simulink model "DirectionFinder"  (R2022b)
settings: Solver=VariableStepAuto  StartTime=0.0  StopTime=GV.SimTime  FixedStep=Pulse/2  RelTol=1e-3
values from neighbouring files (symbols this model uses):
  GV = GlobalVar    [RunDirectionFinder.m]
undefined symbols (not defined in the file or in its folder): S
libraries: dspswit3 x15, simrfV2elements x9, simrfV2util1 x9, dspstat3 x4, spsBistableLib x2, commrflib2 x2
settings Model: Creator=1NR_Operator_34  LastModifiedBy=1NR_Operator_34

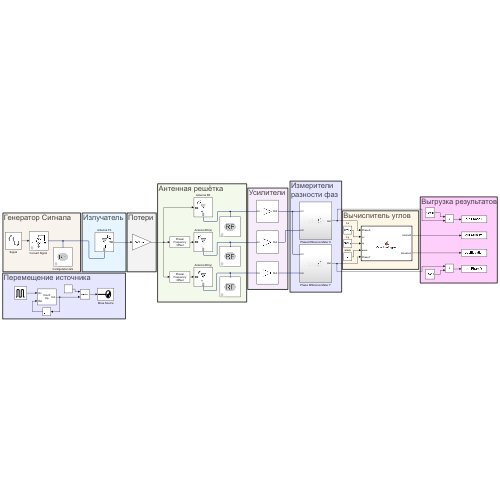
[thumbnail: Simulink's stored preview of the top-level diagram]
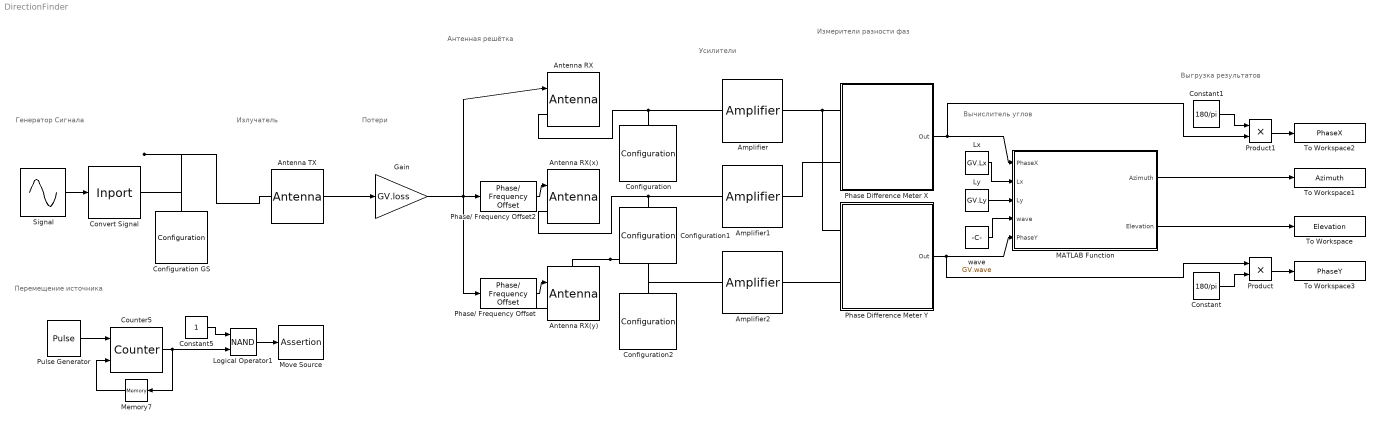
== system DirectionFinder ==
  note: Перемещение источника
  note: Измерители
      | разности фаз
  note: Антенная решётка
  note: Потери
  note: Излучатель
  note: Выгрузка результатов
  note: Вычислитель углов
  note: Усилители
  note: Генератор Сигнала
  Amplifier : simrfV2elements/Amplifier  classname=amplifier  DataSource=Data file  File=unitygain.s2p  isNetworkObj=off  Paramtype=S-parameters  Sparam=[0 0;1 0]  SparamFreq=1e9 Hz  SparamZ0=50  isRationalObj=off  Residues=0  Poles=0  DF={0 0; 1 0}  Source_linear_gain=Available power gain  linear_gain=GV.factor dB  AmAmAmPmTable=[-25,5,-1;-10,20,-2;0,27,5;5,28,12]  Zin=50  Zout=50  Source_Poly=Even and odd order  Poly_Coeffs=[0 1]  IPType=Output  IP2=inf dBm  IP3=inf dBm  P1dB=inf dBm  Psat=inf dBm  Gcomp=inf dBm  InternalGrounding=on  SourceFreq=Extracted from data source  PlotFreq=[1e9:1e6:3e9] Hz  PlotType=X-Y plane  YParam1=S(1,1)  YFormat1=Magnitude (dB)  YParam2=None  YFormat2=Magnitude (dB)  YOption=Linear  XOption=Linear  SparamRepresentation=Time domain (rationalfit)  FitTol=-40  FitOpt=Fit individually  MaxPoles=48  AutoImpulseLength=on  ImpulseLength=1e-10 s  MagModeling=off  AddNoise=on  NoiseType=Noise figure  NoiseDist=White  NF=0  MinNF=0  Gopt=0  RN=0  CarrierFreq=0 Hz  NoiseAutoImpulseLength=on  NoiseImpulseLength=1e-10 s  ConstS21NL=off  OpFreq=1 GHz  SetOpFreqAsMaxS21=off
  Amplifier1 : simrfV2elements/Amplifier  classname=amplifier  DataSource=Data file  File=unitygain.s2p  isNetworkObj=off  Paramtype=S-parameters  Sparam=[0 0;1 0]  SparamFreq=1e9 Hz  SparamZ0=50  isRationalObj=off  Residues=0  Poles=0  DF={0 0; 1 0}  Source_linear_gain=Available power gain  linear_gain=GV.factor dB  AmAmAmPmTable=[-25,5,-1;-10,20,-2;0,27,5;5,28,12]  Zin=50  Zout=50  Source_Poly=Even and odd order  Poly_Coeffs=[0 1]  IPType=Output  IP2=inf dBm  IP3=inf dBm  P1dB=inf dBm  Psat=inf dBm  Gcomp=inf dBm  InternalGrounding=on  SourceFreq=Extracted from data source  PlotFreq=[1e9:1e6:3e9] Hz  PlotType=X-Y plane  YParam1=S(1,1)  YFormat1=Magnitude (dB)  YParam2=None  YFormat2=Magnitude (dB)  YOption=Linear  XOption=Linear  SparamRepresentation=Time domain (rationalfit)  FitTol=-40  FitOpt=Fit individually  MaxPoles=48  AutoImpulseLength=on  ImpulseLength=1e-10 s  MagModeling=off  AddNoise=on  NoiseType=Noise figure  NoiseDist=White  NF=0  MinNF=0  Gopt=0  RN=0  CarrierFreq=0 Hz  NoiseAutoImpulseLength=on  NoiseImpulseLength=1e-10 s  ConstS21NL=off  OpFreq=1 GHz  SetOpFreqAsMaxS21=off
  Amplifier2 : simrfV2elements/Amplifier  classname=amplifier  DataSource=Data file  File=unitygain.s2p  isNetworkObj=off  Paramtype=S-parameters  Sparam=[0 0;1 0]  SparamFreq=1e9 Hz  SparamZ0=50  isRationalObj=off  Residues=0  Poles=0  DF={0 0; 1 0}  Source_linear_gain=Available power gain  linear_gain=GV.factor dB  AmAmAmPmTable=[-25,5,-1;-10,20,-2;0,27,5;5,28,12]  Zin=50  Zout=50  Source_Poly=Even and odd order  Poly_Coeffs=[0 1]  IPType=Output  IP2=inf dBm  IP3=inf dBm  P1dB=inf dBm  Psat=inf dBm  Gcomp=inf dBm  InternalGrounding=on  SourceFreq=Extracted from data source  PlotFreq=[1e9:1e6:3e9] Hz  PlotType=X-Y plane  YParam1=S(1,1)  YFormat1=Magnitude (dB)  YParam2=None  YFormat2=Magnitude (dB)  YOption=Linear  XOption=Linear  SparamRepresentation=Time domain (rationalfit)  FitTol=-40  FitOpt=Fit individually  MaxPoles=48  AutoImpulseLength=on  ImpulseLength=1e-10 s  MagModeling=off  AddNoise=on  NoiseType=Noise figure  NoiseDist=White  NF=0  MinNF=0  Gopt=0  RN=0  CarrierFreq=0 Hz  NoiseAutoImpulseLength=on  NoiseImpulseLength=1e-10 s  ConstS21NL=off  OpFreq=1 GHz  SetOpFreqAsMaxS21=off
  Antenna RX : simrfV2elements/Antenna  AntennaSource=Isotropic radiator  PrevAppliedAntSource=Isotropic radiator  Gr=5 dBi  Zin=50  AntennaObj=AntennaTX  InputIncWave=on  OutputRadWave=off  CarrierFreqInc=GV.freq Hz  rArr=[180 0] deg  CarrierFreqRad=10 Hz  rDep=[0 0] deg  AddNoise=on  InternalGrounding=on  SparamRepresentationImp=Time domain (rationalfit)  FitTolImp=-1  AutoImpulseLengthImp=on  ImpulseLengthImp=1e-10 s
  Antenna RX(x) : simrfV2elements/Antenna  AntennaSource=Isotropic radiator  PrevAppliedAntSource=Isotropic radiator  Gr=5 dBi  Zin=50  AntennaObj=AntennaTX  InputIncWave=on  OutputRadWave=off  CarrierFreqInc=GV.freq Hz  rArr=[180 0] deg  CarrierFreqRad=10 Hz  rDep=[0 0] deg  AddNoise=on  InternalGrounding=on  SparamRepresentationImp=Time domain (rationalfit)  FitTolImp=-1  AutoImpulseLengthImp=on  ImpulseLengthImp=1e-10 s
  Antenna RX(y) : simrfV2elements/Antenna  AntennaSource=Isotropic radiator  PrevAppliedAntSource=Isotropic radiator  Gr=5 dBi  Zin=50  AntennaObj=AntennaTX  InputIncWave=on  OutputRadWave=off  CarrierFreqInc=GV.freq Hz  rArr=[180 0] deg  CarrierFreqRad=10 Hz  rDep=[0 0] deg  AddNoise=on  InternalGrounding=on  SparamRepresentationImp=Time domain (rationalfit)  FitTolImp=-1  AutoImpulseLengthImp=on  ImpulseLengthImp=1e-10 s
  Antenna TX : simrfV2elements/Antenna  AntennaSource=Isotropic radiator  PrevAppliedAntSource=Isotropic radiator  Gr=5 dBi  Zin=50  AntennaObj=AntennaTX  InputIncWave=off  OutputRadWave=on  CarrierFreqInc=2.1 GHz  rArr=[180 0] deg  CarrierFreqRad=GV.freq Hz  rDep=[0 0] deg  AddNoise=on  InternalGrounding=on  SparamRepresentationImp=Time domain (rationalfit)  FitTolImp=-1  AutoImpulseLengthImp=on  ImpulseLengthImp=1e-10 s
  Configuration : simrfV2util1/Configuration  AutoFreq=on  Tones=[433] MHz  Harmonics=[7]  NormalizeCarrierPower=on  SolverType=Auto  UseCCode=on  StepSize=GV.SimStep s  AddNoise=on  defaultRNG=on  Seed=0  Temperature=290.0 K  SolverDelFlag=0  AbsTol=1e-6  RelTol=1e-3  MaxIter=10  ErrorEstimationType=2-norm over all variables  EnableInterpFilter=on  HiddenFIRfilterControllerParam=on  SmallSignalApprox=off  AllSimFreqs=on  SimFreqs=[] Hz  SimFreqsInternal=[]  SamplesPerFrame=1
  Configuration GS : simrfV2util1/Configuration  AutoFreq=on  Tones=[433] MHz  Harmonics=[7]  NormalizeCarrierPower=on  SolverType=Auto  UseCCode=on  StepSize=GV.SimStep s  AddNoise=on  defaultRNG=on  Seed=0  Temperature=290.0 K  SolverDelFlag=0  AbsTol=1e-6  RelTol=1e-3  MaxIter=10  ErrorEstimationType=2-norm over all variables  EnableInterpFilter=on  HiddenFIRfilterControllerParam=on  SmallSignalApprox=off  AllSimFreqs=on  SimFreqs=[] Hz  SimFreqsInternal=[]  SamplesPerFrame=1
  Configuration1 : simrfV2util1/Configuration  AutoFreq=on  Tones=[433] MHz  Harmonics=[7]  NormalizeCarrierPower=on  SolverType=Auto  UseCCode=on  StepSize=GV.SimStep s  AddNoise=on  defaultRNG=on  Seed=0  Temperature=290.0 K  SolverDelFlag=0  AbsTol=1e-6  RelTol=1e-3  MaxIter=10  ErrorEstimationType=2-norm over all variables  EnableInterpFilter=on  HiddenFIRfilterControllerParam=on  SmallSignalApprox=off  AllSimFreqs=on  SimFreqs=[] Hz  SimFreqsInternal=[]  SamplesPerFrame=1
  Configuration2 : simrfV2util1/Configuration  AutoFreq=on  Tones=[433] MHz  Harmonics=[7]  NormalizeCarrierPower=on  SolverType=Auto  UseCCode=on  StepSize=GV.SimStep s  AddNoise=on  defaultRNG=on  Seed=0  Temperature=290.0 K  SolverDelFlag=0  AbsTol=1e-6  RelTol=1e-3  MaxIter=10  ErrorEstimationType=2-norm over all variables  EnableInterpFilter=on  HiddenFIRfilterControllerParam=on  SmallSignalApprox=off  AllSimFreqs=on  SimFreqs=[] Hz  SimFreqsInternal=[]  SamplesPerFrame=1
  Constant : Constant  Value=180/pi
  Constant1 : Constant  Value=180/pi
  Constant5 : Constant
  "Convert Signal " : simrfV2util1/Inport  SimulinkInputSignalType=Ideal voltage  CarrierFreq=GV.freq Hz  ZS=0  UseSqWave=off  NumCoeff=10  Bias=0  DutyCyc=50  InternalGrounding=on
  Counter5 : dspswit3/Counter  Direction=Up  CountEvent=Rising edge  CounterSize=User defined  MaxCount=1  InitialCount=0  Output=Count  HitValue=32  ResetInput=on  SamplesPerFrame=1  Ts=1  CntDtype=double  HitDtype=Logical
  Gain : Gain  Gain=GV.loss
  Logical Operator1 : Logic  Operator=NAND  AllPortsSameDT=off  OutDataTypeStr=boolean
  Lx : Constant  Value=GV.Lx
  Ly : Constant  Value=GV.Ly
  MATLAB Function : MATLAB Function  TreatAsAtomicUnit=on
  Memory7 : Memory
  Move Source : Assertion  AssertionFailFcn=MoveSource  StopWhenAssertionFail=off
  Phase Difference Meter X : Subsystem
  Phase Difference Meter Y : Subsystem
  Phase/ Frequency Offset : commrflib2/Phase// Frequency Offset  phaseOffset=GV.PhaseY(GV.MoveStep)  freqPort=off  freqOffset=0
  Phase/ Frequency Offset2 : commrflib2/Phase// Frequency Offset  phaseOffset=GV.PhaseX(GV.MoveStep)  freqPort=off  freqOffset=0
  Product : Product
  Product1 : Product
  Pulse Generator : DiscretePulseGenerator  PulseType=Time based  Period=GV.SimTime  PulseWidth=50
  Signal : Sin  Amplitude=30  Frequency=2*pi*GV.freq  SampleTime=GV.SimStep
  To Workspace : ToWorkspace  VariableName=Elevation  SampleTime=GV.Measure
      settings: Save2DSignal=2-D array (concatenate along first dimension)
  To Workspace1 : ToWorkspace  VariableName=Azimuth  SampleTime=GV.Measure
      settings: Save2DSignal=2-D array (concatenate along first dimension)
  To Workspace2 : ToWorkspace  VariableName=PhaseX  SampleTime=GV.Measure
      settings: Save2DSignal=2-D array (concatenate along first dimension)
  To Workspace3 : ToWorkspace  VariableName=PhaseY  SampleTime=GV.Measure
      settings: Save2DSignal=2-D array (concatenate along first dimension)
  wave : Constant  Value=GV.wave
  wires:
  Antenna TX/1 -> Gain/1
  MATLAB Function/1(Azimuth) -> To Workspace1/1
  MATLAB Function/2(Elevation) -> To Workspace/1
  Product/1 -> To Workspace3/1
  Constant/1 -> Product/2
  Product1/1 -> To Workspace2/1
  Constant1/1 -> Product1/1
  Phase Difference Meter X/1(Out) -> Product1/2, MATLAB Function/1(PhaseX)
  Phase Difference Meter Y/1(Out) -> MATLAB Function/5(PhaseY), Product/1
  Signal/1 -> "Convert Signal "/1
  Lx/1 -> MATLAB Function/2(Lx)
  Ly/1 -> MATLAB Function/3(Ly)
  wave/1 -> MATLAB Function/4(wave)
  Pulse Generator/1 -> Counter5/1
  Counter5/1 -> Memory7/1, Logical Operator1/2
  Memory7/1 -> Counter5/2
  Constant5/1 -> Logical Operator1/1
  Logical Operator1/1 -> Move Source/1
  Gain/1 -> Antenna RX/1, Phase/ Frequency Offset2/1, Phase/ Frequency Offset/1
  Phase/ Frequency Offset/1 -> Antenna RX(y)/1
  Phase/ Frequency Offset2/1 -> Antenna RX(x)/1
  connections:
  Antenna TX/LConn1 -- "Convert Signal "/RConn1 -- Configuration GS/LConn1
  Amplifier/RConn1 -- Phase Difference Meter Y/LConn1 -- Phase Difference Meter X/LConn1
  Phase Difference Meter X/LConn2 -- Amplifier1/RConn1
  Phase Difference Meter Y/LConn2 -- Amplifier2/RConn1
  Antenna RX(y)/LConn1 -- Amplifier2/LConn1 -- Configuration2/LConn1
  Configuration1/LConn1 -- Amplifier1/LConn1 -- Antenna RX(x)/LConn1
  Configuration/LConn1 -- Amplifier/LConn1 -- Antenna RX/LConn1

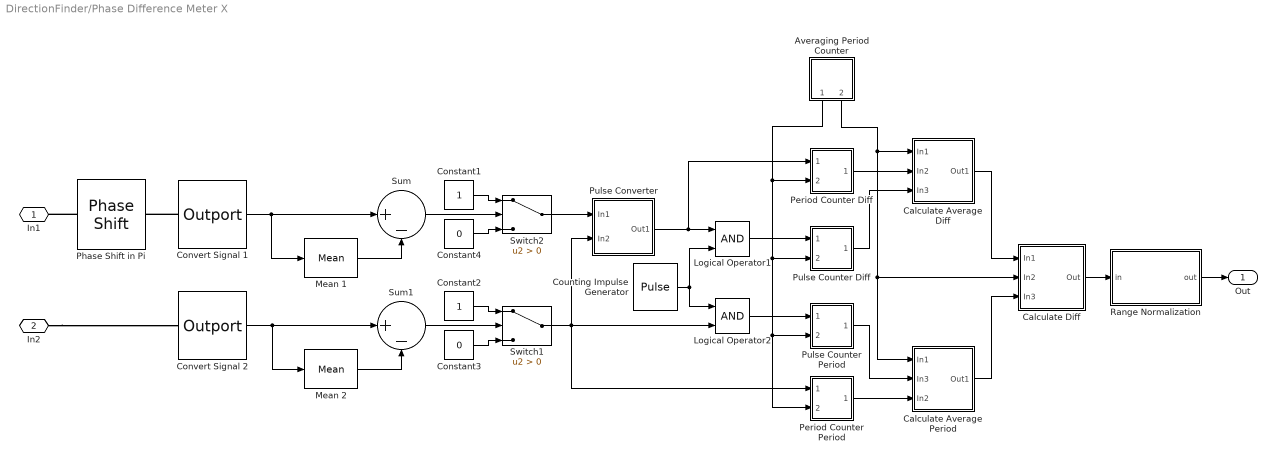
== system DirectionFinder/Phase Difference Meter X ==
  Averaging Period Counter : Subsystem
  Calculate Average Diff : Subsystem
  Calculate Average Period : Subsystem
  Calculate Diff : Subsystem
  Constant1 : Constant
  Constant2 : Constant
  Constant3 : Constant  Value=0
  Constant4 : Constant  Value=0
  Convert Signal 1 : simrfV2util1/Outport  SensorType=Ideal voltage  OutputFormat=Real Passband  CarrierFreq=GV.freq Hz  ZL=Inf  InternalGrounding=on  StepSize=2.3095e-12 s  AutoStep=on
  Convert Signal 2 : simrfV2util1/Outport  SensorType=Ideal voltage  OutputFormat=Real Passband  CarrierFreq=GV.freq Hz  ZL=Inf  InternalGrounding=on  StepSize=2.3095e-12 s  AutoStep=on
  Counting Impulse Generator : DiscretePulseGenerator  PulseType=Time based  Period=GV.Impulse  PulseWidth=50
  Logical Operator1 : Logic  AllPortsSameDT=off  OutDataTypeStr=boolean
  Logical Operator2 : Logic  AllPortsSameDT=off  OutDataTypeStr=boolean
  Mean 1 : dspstat3/Mean  run=on  InputProcessing=Columns as channels (frame based)  reset_popup=None  directionMode=Each column  dimension=1  roiEnable=off  roiType=Rectangles  roiPortion=Entire ROI  roiOutput=Individual statistics for each ROI  roiFlag=off  roundingMode=Floor  overflowMode=off  outputDataTypeStr=Inherit: Same as accumulator  outputMin=[]  outputMax=[]  outputLastDataTypeStr=Inherit: Same as accumulator
  Mean 2 : dspstat3/Mean  run=on  InputProcessing=Columns as channels (frame based)  reset_popup=None  directionMode=Each column  dimension=1  roiEnable=off  roiType=Rectangles  roiPortion=Entire ROI  roiOutput=Individual statistics for each ROI  roiFlag=off  roundingMode=Floor  overflowMode=off  outputDataTypeStr=Inherit: Same as accumulator  outputMin=[]  outputMax=[]  outputLastDataTypeStr=Inherit: Same as accumulator
  Period Counter Diff : Subsystem
  Period Counter Period : Subsystem
  Phase Shift in Pi : simrfV2elements/Phase Shift  PhaseShift=180 deg  InternalGrounding=on
  Pulse Converter : Subsystem
  Pulse Counter Diff : Subsystem
  Pulse Counter Period : Subsystem
  Range Normalization : MATLAB Function  TreatAsAtomicUnit=on
  Sum : Sum  Inputs=|+-
  Sum1 : Sum  Inputs=|+-
  Switch1 : Switch  Criteria=u2 > Threshold  SaturateOnIntegerOverflow=off  InputSameDT=off
  Switch2 : Switch  Criteria=u2 > Threshold  SaturateOnIntegerOverflow=off  InputSameDT=off
  In1 : PMIOPort  Side=Left
  In2 : PMIOPort  Port=2  Side=Left
  Out : Outport
  wires:
  Period Counter Diff/1(Out1) -> Calculate Average Diff/2(In2)
  Averaging Period Counter/1(Out1) -> Period Counter Period/2(In2), Pulse Counter Period/2(In2), Pulse Counter Diff/2(In2), Period Counter Diff/2(In2)
  Sum1/1 -> Switch1/2
  Calculate Average Period/1(Out1) -> Calculate Diff/3(In3)
  Pulse Counter Period/1(Out1) -> Calculate Average Period/2(In3)
  Counting Impulse Generator/1 -> Logical Operator1/2, Logical Operator2/1
  Mean 2/1 -> Sum1/2
  Convert Signal 1/1 -> Mean 1/1, Sum/1
  Mean 1/1 -> Sum/2
  Pulse Counter Diff/1(Out1) -> Calculate Average Diff/3(In3)
  Averaging Period Counter/2(Out2) -> Calculate Average Period/1(In1), Calculate Diff/2(In2), Calculate Average Diff/1(In1)
  Convert Signal 2/1 -> Mean 2/1, Sum1/1
  Logical Operator1/1 -> Pulse Counter Diff/1(In1)
  Calculate Average Diff/1(Out1) -> Calculate Diff/1(In1)
  Period Counter Period/1(Out1) -> Calculate Average Period/3(In2)
  Logical Operator2/1 -> Pulse Counter Period/1(In1)
  Switch2/1 -> Pulse Converter/1(In1)
  Switch1/1 -> Logical Operator2/2, Period Counter Period/1(In1), Pulse Converter/2(In2)
  Pulse Converter/1(Out1) -> Logical Operator1/1, Period Counter Diff/1(In1)
  Calculate Diff/1(Out) -> Range Normalization/1(in)
  Range Normalization/1(out) -> Out/1
  Constant2/1 -> Switch1/1
  Constant3/1 -> Switch1/3
  Sum/1 -> Switch2/2
  Constant1/1 -> Switch2/1
  Constant4/1 -> Switch2/3
  connections:
  In2/RConn1 -- Convert Signal 2/LConn1
  Convert Signal 1/LConn1 -- Phase Shift in Pi/RConn1
  Phase Shift in Pi/LConn1 -- In1/RConn1

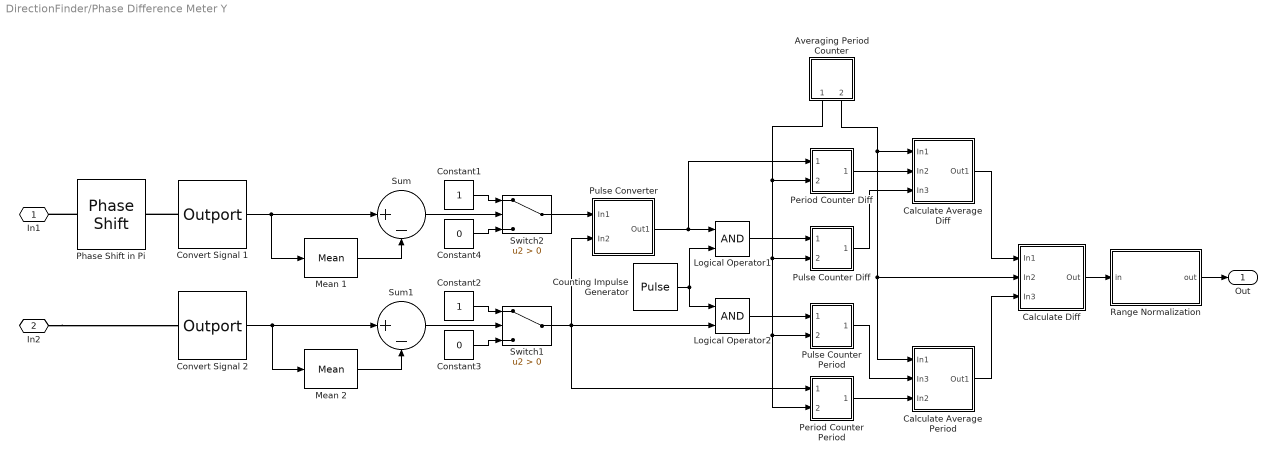
== system DirectionFinder/Phase Difference Meter Y ==
  Averaging Period Counter : Subsystem
  Calculate Average Diff : Subsystem
  Calculate Average Period : Subsystem
  Calculate Diff : Subsystem
  Constant1 : Constant
  Constant2 : Constant
  Constant3 : Constant  Value=0
  Constant4 : Constant  Value=0
  Convert Signal 1 : simrfV2util1/Outport  SensorType=Ideal voltage  OutputFormat=Real Passband  CarrierFreq=GV.freq Hz  ZL=Inf  InternalGrounding=on  StepSize=2.3095e-12 s  AutoStep=on
  Convert Signal 2 : simrfV2util1/Outport  SensorType=Ideal voltage  OutputFormat=Real Passband  CarrierFreq=GV.freq Hz  ZL=Inf  InternalGrounding=on  StepSize=2.3095e-12 s  AutoStep=on
  Counting Impulse Generator : DiscretePulseGenerator  PulseType=Time based  Period=GV.Impulse  PulseWidth=50
  Logical Operator1 : Logic  AllPortsSameDT=off  OutDataTypeStr=boolean
  Logical Operator2 : Logic  AllPortsSameDT=off  OutDataTypeStr=boolean
  Mean 1 : dspstat3/Mean  run=on  InputProcessing=Columns as channels (frame based)  reset_popup=None  directionMode=Each column  dimension=1  roiEnable=off  roiType=Rectangles  roiPortion=Entire ROI  roiOutput=Individual statistics for each ROI  roiFlag=off  roundingMode=Floor  overflowMode=off  outputDataTypeStr=Inherit: Same as accumulator  outputMin=[]  outputMax=[]  outputLastDataTypeStr=Inherit: Same as accumulator
  Mean 2 : dspstat3/Mean  run=on  InputProcessing=Columns as channels (frame based)  reset_popup=None  directionMode=Each column  dimension=1  roiEnable=off  roiType=Rectangles  roiPortion=Entire ROI  roiOutput=Individual statistics for each ROI  roiFlag=off  roundingMode=Floor  overflowMode=off  outputDataTypeStr=Inherit: Same as accumulator  outputMin=[]  outputMax=[]  outputLastDataTypeStr=Inherit: Same as accumulator
  Period Counter Diff : Subsystem
  Period Counter Period : Subsystem
  Phase Shift in Pi : simrfV2elements/Phase Shift  PhaseShift=180 deg  InternalGrounding=on
  Pulse Converter : Subsystem
  Pulse Counter Diff : Subsystem
  Pulse Counter Period : Subsystem
  Range Normalization : MATLAB Function  TreatAsAtomicUnit=on
  Sum : Sum  Inputs=|+-
  Sum1 : Sum  Inputs=|+-
  Switch1 : Switch  Criteria=u2 > Threshold  SaturateOnIntegerOverflow=off  InputSameDT=off
  Switch2 : Switch  Criteria=u2 > Threshold  SaturateOnIntegerOverflow=off  InputSameDT=off
  In1 : PMIOPort  Side=Left
  In2 : PMIOPort  Port=2  Side=Left
  Out : Outport
  wires:
  Period Counter Diff/1(Out1) -> Calculate Average Diff/2(In2)
  Averaging Period Counter/1(Out1) -> Period Counter Period/2(In2), Pulse Counter Period/2(In2), Pulse Counter Diff/2(In2), Period Counter Diff/2(In2)
  Sum1/1 -> Switch1/2
  Calculate Average Period/1(Out1) -> Calculate Diff/3(In3)
  Pulse Counter Period/1(Out1) -> Calculate Average Period/2(In3)
  Counting Impulse Generator/1 -> Logical Operator1/2, Logical Operator2/1
  Mean 2/1 -> Sum1/2
  Convert Signal 1/1 -> Mean 1/1, Sum/1
  Mean 1/1 -> Sum/2
  Pulse Counter Diff/1(Out1) -> Calculate Average Diff/3(In3)
  Averaging Period Counter/2(Out2) -> Calculate Average Period/1(In1), Calculate Diff/2(In2), Calculate Average Diff/1(In1)
  Convert Signal 2/1 -> Mean 2/1, Sum1/1
  Logical Operator1/1 -> Pulse Counter Diff/1(In1)
  Calculate Average Diff/1(Out1) -> Calculate Diff/1(In1)
  Period Counter Period/1(Out1) -> Calculate Average Period/3(In2)
  Logical Operator2/1 -> Pulse Counter Period/1(In1)
  Switch2/1 -> Pulse Converter/1(In1)
  Switch1/1 -> Logical Operator2/2, Period Counter Period/1(In1), Pulse Converter/2(In2)
  Pulse Converter/1(Out1) -> Logical Operator1/1, Period Counter Diff/1(In1)
  Calculate Diff/1(Out) -> Range Normalization/1(in)
  Range Normalization/1(out) -> Out/1
  Constant2/1 -> Switch1/1
  Constant3/1 -> Switch1/3
  Sum/1 -> Switch2/2
  Constant1/1 -> Switch2/1
  Constant4/1 -> Switch2/3
  connections:
  In2/RConn1 -- Convert Signal 2/LConn1
  Convert Signal 1/LConn1 -- Phase Shift in Pi/RConn1
  Phase Shift in Pi/LConn1 -- In1/RConn1

== system DirectionFinder/Phase Difference Meter X/Averaging Period Counter ==
  Constant1 : Constant
  Counter6 : dspswit3/Counter  Direction=Up  CountEvent=Rising edge  CounterSize=User defined  MaxCount=1  InitialCount=0  Output=Count  HitValue=32  ResetInput=on  SamplesPerFrame=1  Ts=1  CntDtype=double  HitDtype=Logical
  Delay : Delay  DelayLength=1  InitialCondition=0
  Logical Operator7 : Logic  Operator=NAND  AllPortsSameDT=off  OutDataTypeStr=boolean
  Measure Period Generator : DiscretePulseGenerator  PulseType=Time based  Period=GV.Measure  PulseWidth=50
  Memory : Memory
  Out1 : Outport
  Out2 : Outport  Port=2
  wires:
  Delay/1 -> Out1/1
  Logical Operator7/1 -> Delay/1
  Measure Period Generator/1 -> Counter6/1
  Counter6/1 -> Memory/1, Out2/1, Logical Operator7/2
  Memory/1 -> Counter6/2
  Constant1/1 -> Logical Operator7/1

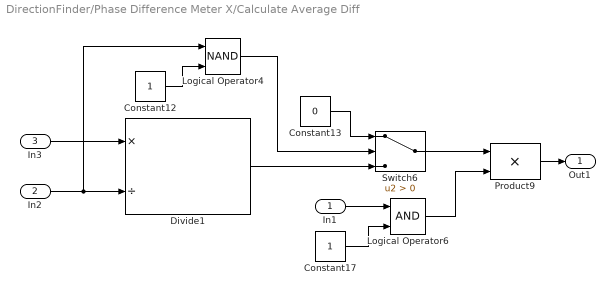
== system DirectionFinder/Phase Difference Meter X/Calculate Average Diff ==
  In1 : Inport
  In2 : Inport  Port=2
  In3 : Inport  Port=3
  Constant12 : Constant
  Constant13 : Constant  Value=0
  Constant17 : Constant
  Divide1 : Product  Inputs=*/
  Logical Operator4 : Logic  Operator=NAND  AllPortsSameDT=off  OutDataTypeStr=boolean
  Logical Operator6 : Logic  AllPortsSameDT=off  OutDataTypeStr=boolean
  Product9 : Product
  Switch6 : Switch  Criteria=u2 > Threshold  SaturateOnIntegerOverflow=off  InputSameDT=off
  Out1 : Outport
  wires:
  Divide1/1 -> Switch6/3
  Logical Operator6/1 -> Product9/2
  Constant17/1 -> Logical Operator6/2
  Constant12/1 -> Logical Operator4/2
  Logical Operator4/1 -> Switch6/2
  Constant13/1 -> Switch6/1
  Switch6/1 -> Product9/1
  In2/1 -> Logical Operator4/1, Divide1/2
  Product9/1 -> Out1/1
  In1/1 -> Logical Operator6/1
  In3/1 -> Divide1/1

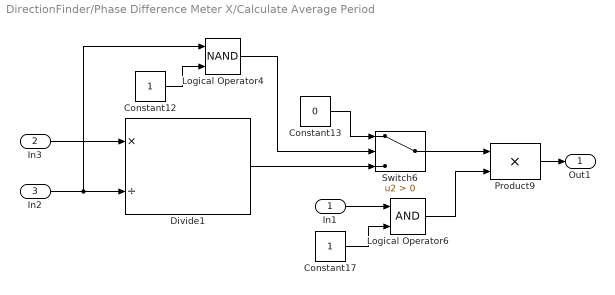
== system DirectionFinder/Phase Difference Meter X/Calculate Average Period ==
  In1 : Inport
  In3 : Inport  Port=2
  In2 : Inport  Port=3
  Constant12 : Constant
  Constant13 : Constant  Value=0
  Constant17 : Constant
  Divide1 : Product  Inputs=*/
  Logical Operator4 : Logic  Operator=NAND  AllPortsSameDT=off  OutDataTypeStr=boolean
  Logical Operator6 : Logic  AllPortsSameDT=off  OutDataTypeStr=boolean
  Product9 : Product
  Switch6 : Switch  Criteria=u2 > Threshold  SaturateOnIntegerOverflow=off  InputSameDT=off
  Out1 : Outport
  wires:
  Divide1/1 -> Switch6/3
  Logical Operator6/1 -> Product9/2
  Constant17/1 -> Logical Operator6/2
  Constant12/1 -> Logical Operator4/2
  Logical Operator4/1 -> Switch6/2
  Constant13/1 -> Switch6/1
  Switch6/1 -> Product9/1
  In2/1 -> Logical Operator4/1, Divide1/2
  Product9/1 -> Out1/1
  In1/1 -> Logical Operator6/1
  In3/1 -> Divide1/1

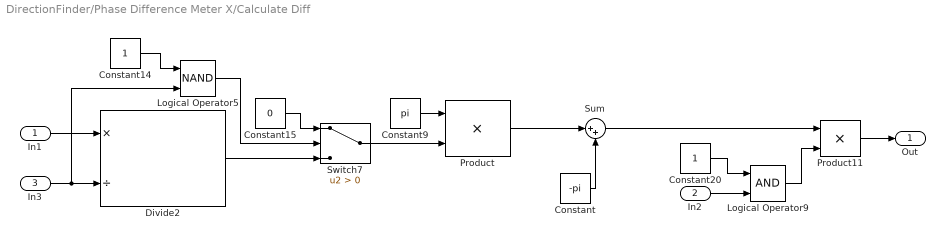
== system DirectionFinder/Phase Difference Meter X/Calculate Diff ==
  In1 : Inport
  In2 : Inport  Port=2
  In3 : Inport  Port=3
  Constant : Constant  Value=-pi
  Constant14 : Constant
  Constant15 : Constant  Value=0
  Constant20 : Constant
  Constant9 : Constant  Value=pi
  Divide2 : Product  Inputs=*/
  Logical Operator5 : Logic  Operator=NAND  AllPortsSameDT=off  OutDataTypeStr=boolean
  Logical Operator9 : Logic  AllPortsSameDT=off  OutDataTypeStr=boolean
  Product : Product
  Product11 : Product
  Sum : Sum  Inputs=|++
  Switch7 : Switch  Criteria=u2 > Threshold  SaturateOnIntegerOverflow=off  InputSameDT=off
  Out : Outport
  wires:
  Constant9/1 -> Product/1
  Divide2/1 -> Switch7/3
  Logical Operator5/1 -> Switch7/2
  In3/1 -> Logical Operator5/2, Divide2/2
  Switch7/1 -> Product/2
  Constant15/1 -> Switch7/1
  Logical Operator9/1 -> Product11/2
  Product11/1 -> Out/1
  In1/1 -> Divide2/1
  Constant14/1 -> Logical Operator5/1
  Constant20/1 -> Logical Operator9/1
  In2/1 -> Logical Operator9/2
  Constant/1 -> Sum/2
  Product/1 -> Sum/1
  Sum/1 -> Product11/1

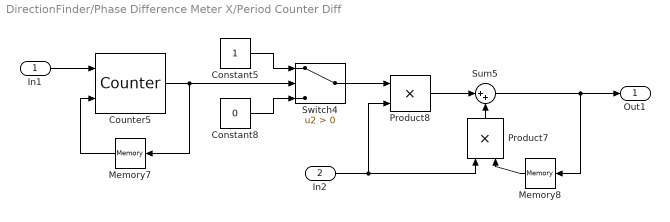
== system DirectionFinder/Phase Difference Meter X/Period Counter Diff ==
  In1 : Inport
  In2 : Inport  Port=2
  Constant5 : Constant
  Constant8 : Constant  Value=0
  Counter5 : dspswit3/Counter  Direction=Up  CountEvent=Rising edge  CounterSize=User defined  MaxCount=1  InitialCount=0  Output=Count  HitValue=32  ResetInput=on  SamplesPerFrame=1  Ts=1  CntDtype=double  HitDtype=Logical
  Memory7 : Memory
  Memory8 : Memory
  Product7 : Product
  Product8 : Product
  Sum5 : Sum  Inputs=|++
  Switch4 : Switch  Criteria=u2 > Threshold  SaturateOnIntegerOverflow=off  InputSameDT=off
  Out1 : Outport
  wires:
  Counter5/1 -> Memory7/1, Switch4/2
  Product8/1 -> Sum5/1
  Switch4/1 -> Product8/1
  Constant5/1 -> Switch4/1
  Sum5/1 -> Out1/1, Memory8/1
  Memory8/1 -> Product7/2
  Constant8/1 -> Switch4/3
  Memory7/1 -> Counter5/2
  In2/1 -> Product7/1, Product8/2
  Product7/1 -> Sum5/2
  In1/1 -> Counter5/1

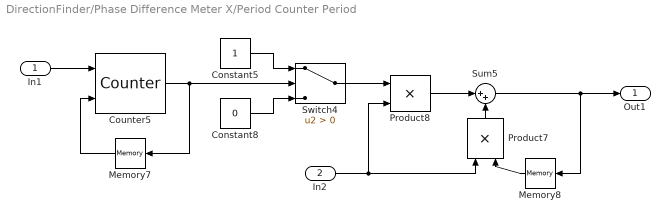
== system DirectionFinder/Phase Difference Meter X/Period Counter Period ==
  In1 : Inport
  In2 : Inport  Port=2
  Constant5 : Constant
  Constant8 : Constant  Value=0
  Counter5 : dspswit3/Counter  Direction=Up  CountEvent=Rising edge  CounterSize=User defined  MaxCount=1  InitialCount=0  Output=Count  HitValue=32  ResetInput=on  SamplesPerFrame=1  Ts=1  CntDtype=double  HitDtype=Logical
  Memory7 : Memory
  Memory8 : Memory
  Product7 : Product
  Product8 : Product
  Sum5 : Sum  Inputs=|++
  Switch4 : Switch  Criteria=u2 > Threshold  SaturateOnIntegerOverflow=off  InputSameDT=off
  Out1 : Outport
  wires:
  Counter5/1 -> Memory7/1, Switch4/2
  Product8/1 -> Sum5/1
  Switch4/1 -> Product8/1
  Constant5/1 -> Switch4/1
  Sum5/1 -> Out1/1, Memory8/1
  Memory8/1 -> Product7/2
  Constant8/1 -> Switch4/3
  Memory7/1 -> Counter5/2
  In2/1 -> Product7/1, Product8/2
  Product7/1 -> Sum5/2
  In1/1 -> Counter5/1

== system DirectionFinder/Phase Difference Meter X/Pulse Converter ==
  In1 : Inport
  In2 : Inport  Port=2
  Bistable : spsBistableLib/Bistable  Qpriority=Set  ic=0  Ts=0
      settings: LibrarySourceBlock=sps_lib/Control/Bistable
  Counter1 : dspswit3/Counter  Direction=Up  CountEvent=Rising edge  CounterSize=User defined  MaxCount=1  InitialCount=0  Output=Count  HitValue=32  ResetInput=on  SamplesPerFrame=1  Ts=1  CntDtype=double  HitDtype=Logical
  Counter5 : dspswit3/Counter  Direction=Up  CountEvent=Rising edge  CounterSize=User defined  MaxCount=1  InitialCount=0  Output=Count  HitValue=32  ResetInput=on  SamplesPerFrame=1  Ts=1  CntDtype=double  HitDtype=Logical
  Memory1 : Memory
  Memory7 : Memory
  Terminator : Terminator
  Out1 : Outport
  wires:
  Memory7/1 -> Counter5/2
  Counter5/1 -> Memory7/1, Bistable/1
  In1/1 -> Counter5/1
  In2/1 -> Counter1/1
  Counter1/1 -> Bistable/2, Memory1/1
  Memory1/1 -> Counter1/2
  Bistable/1 -> Terminator/1
  Bistable/2 -> Out1/1

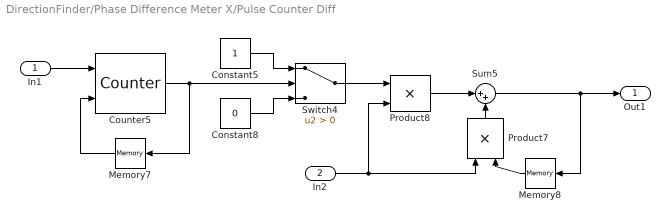
== system DirectionFinder/Phase Difference Meter X/Pulse Counter Diff ==
  In1 : Inport
  In2 : Inport  Port=2
  Constant5 : Constant
  Constant8 : Constant  Value=0
  Counter5 : dspswit3/Counter  Direction=Up  CountEvent=Rising edge  CounterSize=User defined  MaxCount=1  InitialCount=0  Output=Count  HitValue=32  ResetInput=on  SamplesPerFrame=1  Ts=1  CntDtype=double  HitDtype=Logical
  Memory7 : Memory
  Memory8 : Memory
  Product7 : Product
  Product8 : Product
  Sum5 : Sum  Inputs=|++
  Switch4 : Switch  Criteria=u2 > Threshold  SaturateOnIntegerOverflow=off  InputSameDT=off
  Out1 : Outport
  wires:
  Counter5/1 -> Memory7/1, Switch4/2
  Product8/1 -> Sum5/1
  Switch4/1 -> Product8/1
  Constant5/1 -> Switch4/1
  Sum5/1 -> Out1/1, Memory8/1
  Memory8/1 -> Product7/2
  Constant8/1 -> Switch4/3
  Memory7/1 -> Counter5/2
  In2/1 -> Product7/1, Product8/2
  Product7/1 -> Sum5/2
  In1/1 -> Counter5/1

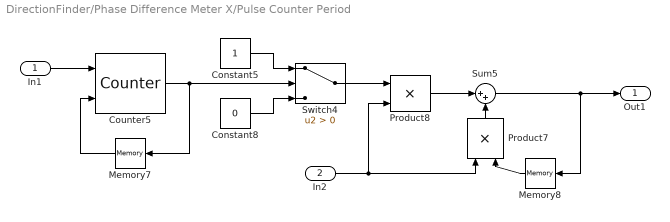
== system DirectionFinder/Phase Difference Meter X/Pulse Counter Period ==
  In1 : Inport
  In2 : Inport  Port=2
  Constant5 : Constant
  Constant8 : Constant  Value=0
  Counter5 : dspswit3/Counter  Direction=Up  CountEvent=Rising edge  CounterSize=User defined  MaxCount=1  InitialCount=0  Output=Count  HitValue=32  ResetInput=on  SamplesPerFrame=1  Ts=1  CntDtype=double  HitDtype=Logical
  Memory7 : Memory
  Memory8 : Memory
  Product7 : Product
  Product8 : Product
  Sum5 : Sum  Inputs=|++
  Switch4 : Switch  Criteria=u2 > Threshold  SaturateOnIntegerOverflow=off  InputSameDT=off
  Out1 : Outport
  wires:
  Counter5/1 -> Memory7/1, Switch4/2
  Product8/1 -> Sum5/1
  Switch4/1 -> Product8/1
  Constant5/1 -> Switch4/1
  Sum5/1 -> Out1/1, Memory8/1
  Memory8/1 -> Product7/2
  Constant8/1 -> Switch4/3
  Memory7/1 -> Counter5/2
  In2/1 -> Product7/1, Product8/2
  Product7/1 -> Sum5/2
  In1/1 -> Counter5/1

== system DirectionFinder/Phase Difference Meter Y/Averaging Period Counter ==
  Constant1 : Constant
  Counter6 : dspswit3/Counter  Direction=Up  CountEvent=Rising edge  CounterSize=User defined  MaxCount=1  InitialCount=0  Output=Count  HitValue=32  ResetInput=on  SamplesPerFrame=1  Ts=1  CntDtype=double  HitDtype=Logical
  Delay : Delay  DelayLength=1  InitialCondition=0
  Logical Operator7 : Logic  Operator=NAND  AllPortsSameDT=off  OutDataTypeStr=boolean
  Measure Period Generator : DiscretePulseGenerator  PulseType=Time based  Period=GV.Measure  PulseWidth=50
  Memory : Memory
  Out1 : Outport
  Out2 : Outport  Port=2
  wires:
  Delay/1 -> Out1/1
  Logical Operator7/1 -> Delay/1
  Measure Period Generator/1 -> Counter6/1
  Counter6/1 -> Memory/1, Out2/1, Logical Operator7/2
  Memory/1 -> Counter6/2
  Constant1/1 -> Logical Operator7/1

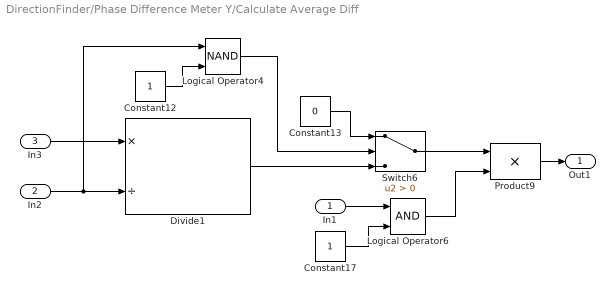
== system DirectionFinder/Phase Difference Meter Y/Calculate Average Diff ==
  In1 : Inport
  In2 : Inport  Port=2
  In3 : Inport  Port=3
  Constant12 : Constant
  Constant13 : Constant  Value=0
  Constant17 : Constant
  Divide1 : Product  Inputs=*/
  Logical Operator4 : Logic  Operator=NAND  AllPortsSameDT=off  OutDataTypeStr=boolean
  Logical Operator6 : Logic  AllPortsSameDT=off  OutDataTypeStr=boolean
  Product9 : Product
  Switch6 : Switch  Criteria=u2 > Threshold  SaturateOnIntegerOverflow=off  InputSameDT=off
  Out1 : Outport
  wires:
  Divide1/1 -> Switch6/3
  Logical Operator6/1 -> Product9/2
  Constant17/1 -> Logical Operator6/2
  Constant12/1 -> Logical Operator4/2
  Logical Operator4/1 -> Switch6/2
  Constant13/1 -> Switch6/1
  Switch6/1 -> Product9/1
  In2/1 -> Logical Operator4/1, Divide1/2
  Product9/1 -> Out1/1
  In1/1 -> Logical Operator6/1
  In3/1 -> Divide1/1

== system DirectionFinder/Phase Difference Meter Y/Calculate Average Period ==
  In1 : Inport
  In3 : Inport  Port=2
  In2 : Inport  Port=3
  Constant12 : Constant
  Constant13 : Constant  Value=0
  Constant17 : Constant
  Divide1 : Product  Inputs=*/
  Logical Operator4 : Logic  Operator=NAND  AllPortsSameDT=off  OutDataTypeStr=boolean
  Logical Operator6 : Logic  AllPortsSameDT=off  OutDataTypeStr=boolean
  Product9 : Product
  Switch6 : Switch  Criteria=u2 > Threshold  SaturateOnIntegerOverflow=off  InputSameDT=off
  Out1 : Outport
  wires:
  Divide1/1 -> Switch6/3
  Logical Operator6/1 -> Product9/2
  Constant17/1 -> Logical Operator6/2
  Constant12/1 -> Logical Operator4/2
  Logical Operator4/1 -> Switch6/2
  Constant13/1 -> Switch6/1
  Switch6/1 -> Product9/1
  In2/1 -> Logical Operator4/1, Divide1/2
  Product9/1 -> Out1/1
  In1/1 -> Logical Operator6/1
  In3/1 -> Divide1/1

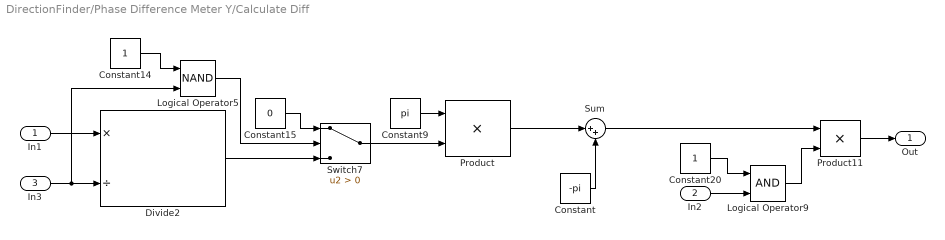
== system DirectionFinder/Phase Difference Meter Y/Calculate Diff ==
  In1 : Inport
  In2 : Inport  Port=2
  In3 : Inport  Port=3
  Constant : Constant  Value=-pi
  Constant14 : Constant
  Constant15 : Constant  Value=0
  Constant20 : Constant
  Constant9 : Constant  Value=pi
  Divide2 : Product  Inputs=*/
  Logical Operator5 : Logic  Operator=NAND  AllPortsSameDT=off  OutDataTypeStr=boolean
  Logical Operator9 : Logic  AllPortsSameDT=off  OutDataTypeStr=boolean
  Product : Product
  Product11 : Product
  Sum : Sum  Inputs=|++
  Switch7 : Switch  Criteria=u2 > Threshold  SaturateOnIntegerOverflow=off  InputSameDT=off
  Out : Outport
  wires:
  Constant9/1 -> Product/1
  Divide2/1 -> Switch7/3
  Logical Operator5/1 -> Switch7/2
  In3/1 -> Logical Operator5/2, Divide2/2
  Switch7/1 -> Product/2
  Constant15/1 -> Switch7/1
  Logical Operator9/1 -> Product11/2
  Product11/1 -> Out/1
  In1/1 -> Divide2/1
  Constant14/1 -> Logical Operator5/1
  Constant20/1 -> Logical Operator9/1
  In2/1 -> Logical Operator9/2
  Constant/1 -> Sum/2
  Product/1 -> Sum/1
  Sum/1 -> Product11/1

== system DirectionFinder/Phase Difference Meter Y/Period Counter Diff ==
  In1 : Inport
  In2 : Inport  Port=2
  Constant5 : Constant
  Constant8 : Constant  Value=0
  Counter5 : dspswit3/Counter  Direction=Up  CountEvent=Rising edge  CounterSize=User defined  MaxCount=1  InitialCount=0  Output=Count  HitValue=32  ResetInput=on  SamplesPerFrame=1  Ts=1  CntDtype=double  HitDtype=Logical
  Memory7 : Memory
  Memory8 : Memory
  Product7 : Product
  Product8 : Product
  Sum5 : Sum  Inputs=|++
  Switch4 : Switch  Criteria=u2 > Threshold  SaturateOnIntegerOverflow=off  InputSameDT=off
  Out1 : Outport
  wires:
  Counter5/1 -> Memory7/1, Switch4/2
  Product8/1 -> Sum5/1
  Switch4/1 -> Product8/1
  Constant5/1 -> Switch4/1
  Sum5/1 -> Out1/1, Memory8/1
  Memory8/1 -> Product7/2
  Constant8/1 -> Switch4/3
  Memory7/1 -> Counter5/2
  In2/1 -> Product7/1, Product8/2
  Product7/1 -> Sum5/2
  In1/1 -> Counter5/1

== system DirectionFinder/Phase Difference Meter Y/Period Counter Period ==
  In1 : Inport
  In2 : Inport  Port=2
  Constant5 : Constant
  Constant8 : Constant  Value=0
  Counter5 : dspswit3/Counter  Direction=Up  CountEvent=Rising edge  CounterSize=User defined  MaxCount=1  InitialCount=0  Output=Count  HitValue=32  ResetInput=on  SamplesPerFrame=1  Ts=1  CntDtype=double  HitDtype=Logical
  Memory7 : Memory
  Memory8 : Memory
  Product7 : Product
  Product8 : Product
  Sum5 : Sum  Inputs=|++
  Switch4 : Switch  Criteria=u2 > Threshold  SaturateOnIntegerOverflow=off  InputSameDT=off
  Out1 : Outport
  wires:
  Counter5/1 -> Memory7/1, Switch4/2
  Product8/1 -> Sum5/1
  Switch4/1 -> Product8/1
  Constant5/1 -> Switch4/1
  Sum5/1 -> Out1/1, Memory8/1
  Memory8/1 -> Product7/2
  Constant8/1 -> Switch4/3
  Memory7/1 -> Counter5/2
  In2/1 -> Product7/1, Product8/2
  Product7/1 -> Sum5/2
  In1/1 -> Counter5/1

== system DirectionFinder/Phase Difference Meter Y/Pulse Converter ==
  In1 : Inport
  In2 : Inport  Port=2
  Bistable : spsBistableLib/Bistable  Qpriority=Set  ic=0  Ts=0
      settings: LibrarySourceBlock=sps_lib/Control/Bistable
  Counter1 : dspswit3/Counter  Direction=Up  CountEvent=Rising edge  CounterSize=User defined  MaxCount=1  InitialCount=0  Output=Count  HitValue=32  ResetInput=on  SamplesPerFrame=1  Ts=1  CntDtype=double  HitDtype=Logical
  Counter5 : dspswit3/Counter  Direction=Up  CountEvent=Rising edge  CounterSize=User defined  MaxCount=1  InitialCount=0  Output=Count  HitValue=32  ResetInput=on  SamplesPerFrame=1  Ts=1  CntDtype=double  HitDtype=Logical
  Memory1 : Memory
  Memory7 : Memory
  Terminator : Terminator
  Out1 : Outport
  wires:
  Memory7/1 -> Counter5/2
  Counter5/1 -> Memory7/1, Bistable/1
  In1/1 -> Counter5/1
  In2/1 -> Counter1/1
  Counter1/1 -> Bistable/2, Memory1/1
  Memory1/1 -> Counter1/2
  Bistable/1 -> Terminator/1
  Bistable/2 -> Out1/1

== system DirectionFinder/Phase Difference Meter Y/Pulse Counter Diff ==
  In1 : Inport
  In2 : Inport  Port=2
  Constant5 : Constant
  Constant8 : Constant  Value=0
  Counter5 : dspswit3/Counter  Direction=Up  CountEvent=Rising edge  CounterSize=User defined  MaxCount=1  InitialCount=0  Output=Count  HitValue=32  ResetInput=on  SamplesPerFrame=1  Ts=1  CntDtype=double  HitDtype=Logical
  Memory7 : Memory
  Memory8 : Memory
  Product7 : Product
  Product8 : Product
  Sum5 : Sum  Inputs=|++
  Switch4 : Switch  Criteria=u2 > Threshold  SaturateOnIntegerOverflow=off  InputSameDT=off
  Out1 : Outport
  wires:
  Counter5/1 -> Memory7/1, Switch4/2
  Product8/1 -> Sum5/1
  Switch4/1 -> Product8/1
  Constant5/1 -> Switch4/1
  Sum5/1 -> Out1/1, Memory8/1
  Memory8/1 -> Product7/2
  Constant8/1 -> Switch4/3
  Memory7/1 -> Counter5/2
  In2/1 -> Product7/1, Product8/2
  Product7/1 -> Sum5/2
  In1/1 -> Counter5/1

== system DirectionFinder/Phase Difference Meter Y/Pulse Counter Period ==
  In1 : Inport
  In2 : Inport  Port=2
  Constant5 : Constant
  Constant8 : Constant  Value=0
  Counter5 : dspswit3/Counter  Direction=Up  CountEvent=Rising edge  CounterSize=User defined  MaxCount=1  InitialCount=0  Output=Count  HitValue=32  ResetInput=on  SamplesPerFrame=1  Ts=1  CntDtype=double  HitDtype=Logical
  Memory7 : Memory
  Memory8 : Memory
  Product7 : Product
  Product8 : Product
  Sum5 : Sum  Inputs=|++
  Switch4 : Switch  Criteria=u2 > Threshold  SaturateOnIntegerOverflow=off  InputSameDT=off
  Out1 : Outport
  wires:
  Counter5/1 -> Memory7/1, Switch4/2
  Product8/1 -> Sum5/1
  Switch4/1 -> Product8/1
  Constant5/1 -> Switch4/1
  Sum5/1 -> Out1/1, Memory8/1
  Memory8/1 -> Product7/2
  Constant8/1 -> Switch4/3
  Memory7/1 -> Counter5/2
  In2/1 -> Product7/1, Product8/2
  Product7/1 -> Sum5/2
  In1/1 -> Counter5/1

== matlab function DirectionFinder/Phase Difference Meter Y/Range Normalization ==
  data: in input; out output
function out = Normalization(in)

if in > pi
    out = in - 2*pi;
else
   out = in;
end

end

== matlab function DirectionFinder/MATLAB Function ==
  data: PhaseX input; Lx input; Ly input; wave input; Azimuth output; PhaseY input; Elevation output
function [Azimuth,Elevation] = CalculateAngles(PhaseX,Lx,Ly,wave,PhaseY)

if abs(PhaseX) > (0.3*(pi/180)) % с погрешностью 0.3 градуса
    Azimuth = atan(PhaseY*Lx/(PhaseX*Ly))*180/pi;
else
    Azimuth = 90;
end

arg = wave/(2*pi)*sqrt((PhaseX/Lx)^(2)+(PhaseY/Ly)^(2));

if arg > 1
    Elevation = 0;
else
    Elevation = acos(arg)*180/pi;
end

end

== matlab function DirectionFinder/Phase Difference Meter X/Range Normalization ==
  data: in input; out output
function out = Normalization(in)

if in > pi
    out = in - 2*pi;
else
   out = in;
end

end
